simulink model "UticajSmetnji"  (R2014b)
settings: Solver=ode3  StartTime=0.0  StopTime=300  FixedStep=0.001  RelTol=1e-3
libraries: simulink x7
settings Model: Creator=Korisnik  LastModifiedBy=Korisnik

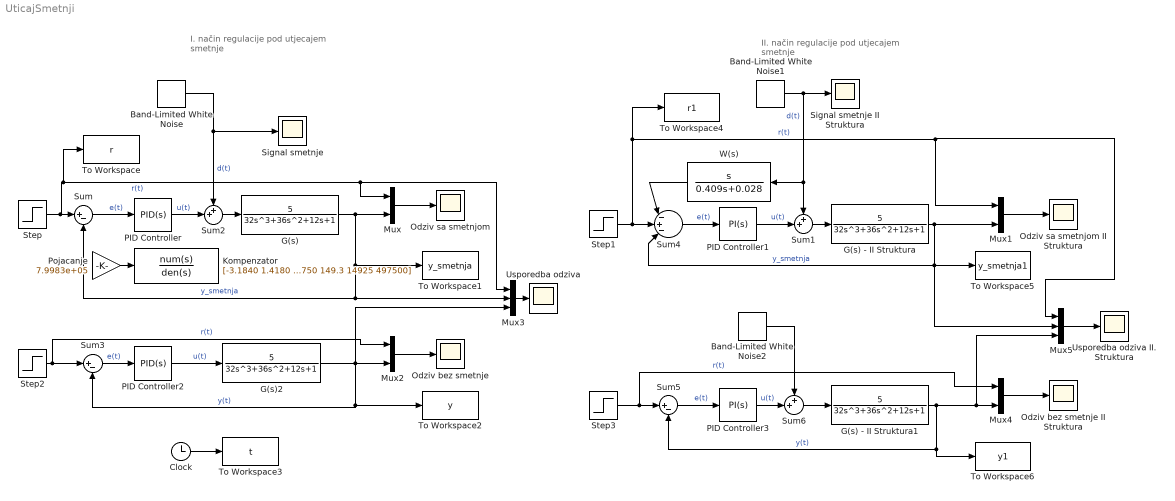
== system UticajSmetnji ==
  note: II. način regulacije pod utjecajem
      |                      smetnje
  note: I. način regulacije pod utjecajem
      |                     smetnje
  Band-Limited White Noise : simulink/Sources/Band-Limited White Noise  Cov=[0.001]  Ts=0.001  seed=[23341]
  Band-Limited White Noise1 : simulink/Sources/Band-Limited White Noise  Cov=[0.001]  Ts=0.001  seed=[23341]
  Band-Limited White Noise2 : simulink/Sources/Band-Limited White Noise  Cov=[0.001]  Ts=0.001  seed=[23341]
  Clock : Clock
  G(s) : TransferFcn  Numerator=[5]  Denominator=[32 36 12 1]
  G(s) - II Struktura : TransferFcn  Numerator=[5]  Denominator=[32 36 12 1]
  G(s) - II Struktura1 : TransferFcn  Numerator=[5]  Denominator=[32 36 12 1]
  G(s)2 : TransferFcn  Numerator=[5]  Denominator=[32 36 12 1]
  Kompenzator : TransferFcn  Numerator=[-3.1840 1.4180 1.0360 0.3980]  Denominator=[4.9750 149.3 14925 497500]
  Mux{,1..2,4} (4 alike) : Mux  Inputs=2
  Mux3 : Mux  Inputs=3
  Mux5 : Mux  Inputs=3
  Odziv bez smetnje : Scope
      settings: ShowLegends=on  SaveName=ScopeData2
  Odziv bez smetnje II Struktura : Scope
      settings: ShowLegends=on  SaveName=ScopeData6
  Odziv sa smetnjom : Scope
      settings: ShowLegends=on
  Odziv sa smetnjom II Struktura : Scope
      settings: ShowLegends=on
  PID Controller : simulink/Continuous/PID Controller  Controller=PID  TimeDomain=Continuous-time  SampleTime=-1  IntegratorMethod=Forward Euler  FilterMethod=Forward Euler  Form=Parallel  P=0.400421573227882  I=0.0460624565194868  D=0.464403326069187  N=2.07495559131807  InitialConditionSource=internal  InitialConditionForIntegrator=0  InitialConditionForFilter=0  ExternalReset=none  LimitOutput=off  UpperSaturationLimit=inf  LowerSaturationLimit=-inf  LinearizeAsGain=on  AntiWindupMode=none  Kb=1  TrackingMode=off  Kt=1  PParamMin=[]  PParamMax=[]  IParamMin=[]  IParamMax=[]  DParamMin=[]  DParamMax=[]  NParamMin=[]  NParamMax=[]  KbParamMin=[]  KbParamMax=[]  KtParamMin=[]  KtParamMax=[]  POutMin=[]  POutMax=[]  IOutMin=[]  IOutMax=[]  DOutMin=[]  DOutMax=[]  NOutMin=[]  NOutMax=[]  KbOutMin=[]  KbOutMax=[]  KtOutMin=[]  KtOutMax=[]  IntegratorOutMin=[]  IntegratorOutMax=[]  FilterOutMin=[]  FilterOutMax=[]  SumOutMin=[]  SumOutMax=[]  SumI1OutMin=[]  SumI1OutMax=[]  SumI2OutMin=[]  SumI2OutMax=[]  SumI3OutMin=[]  SumI3OutMax=[]  SumDOutMin=[]  SumDOutMax=[]  SaturationOutMin=[]  SaturationOutMax=[]  IntegratorContinuousStateAttributes=''  IntegratorStateMustResolveToSignalObject=off  IntegratorRTWStateStorageClass=Auto  FilterContinuousStateAttributes=''  FilterStateMustResolveToSignalObject=off  FilterRTWStateStorageClass=Auto  DifferentiatorICPrevScaledInput=0  DifferentiatorOutMin=[]  DifferentiatorOutMax=[]  UseFilter=on
  PID Controller1 : simulink/Continuous/PID Controller  Controller=PI  TimeDomain=Continuous-time  SampleTime=-1  IntegratorMethod=Forward Euler  FilterMethod=Forward Euler  Form=Parallel  P=0.409  I=0.028  D=0.464403326069187  N=2.07495559131807  InitialConditionSource=internal  InitialConditionForIntegrator=0  InitialConditionForFilter=0  ExternalReset=none  LimitOutput=off  UpperSaturationLimit=inf  LowerSaturationLimit=-inf  LinearizeAsGain=on  AntiWindupMode=none  Kb=1  TrackingMode=off  Kt=1  PParamMin=[]  PParamMax=[]  IParamMin=[]  IParamMax=[]  DParamMin=[]  DParamMax=[]  NParamMin=[]  NParamMax=[]  KbParamMin=[]  KbParamMax=[]  KtParamMin=[]  KtParamMax=[]  POutMin=[]  POutMax=[]  IOutMin=[]  IOutMax=[]  DOutMin=[]  DOutMax=[]  NOutMin=[]  NOutMax=[]  KbOutMin=[]  KbOutMax=[]  KtOutMin=[]  KtOutMax=[]  IntegratorOutMin=[]  IntegratorOutMax=[]  FilterOutMin=[]  FilterOutMax=[]  SumOutMin=[]  SumOutMax=[]  SumI1OutMin=[]  SumI1OutMax=[]  SumI2OutMin=[]  SumI2OutMax=[]  SumI3OutMin=[]  SumI3OutMax=[]  SumDOutMin=[]  SumDOutMax=[]  SaturationOutMin=[]  SaturationOutMax=[]  IntegratorContinuousStateAttributes=''  IntegratorStateMustResolveToSignalObject=off  IntegratorRTWStateStorageClass=Auto  FilterContinuousStateAttributes=''  FilterStateMustResolveToSignalObject=off  FilterRTWStateStorageClass=Auto  DifferentiatorICPrevScaledInput=0  DifferentiatorOutMin=[]  DifferentiatorOutMax=[]  UseFilter=on
  PID Controller2 : simulink/Continuous/PID Controller  Controller=PID  TimeDomain=Continuous-time  SampleTime=-1  IntegratorMethod=Forward Euler  FilterMethod=Forward Euler  Form=Parallel  P=0.400421573227882  I=0.0460624565194868  D=0.464403326069187  N=2.07495559131807  InitialConditionSource=internal  InitialConditionForIntegrator=0  InitialConditionForFilter=0  ExternalReset=none  LimitOutput=off  UpperSaturationLimit=inf  LowerSaturationLimit=-inf  LinearizeAsGain=on  AntiWindupMode=none  Kb=1  TrackingMode=off  Kt=1  PParamMin=[]  PParamMax=[]  IParamMin=[]  IParamMax=[]  DParamMin=[]  DParamMax=[]  NParamMin=[]  NParamMax=[]  KbParamMin=[]  KbParamMax=[]  KtParamMin=[]  KtParamMax=[]  POutMin=[]  POutMax=[]  IOutMin=[]  IOutMax=[]  DOutMin=[]  DOutMax=[]  NOutMin=[]  NOutMax=[]  KbOutMin=[]  KbOutMax=[]  KtOutMin=[]  KtOutMax=[]  IntegratorOutMin=[]  IntegratorOutMax=[]  FilterOutMin=[]  FilterOutMax=[]  SumOutMin=[]  SumOutMax=[]  SumI1OutMin=[]  SumI1OutMax=[]  SumI2OutMin=[]  SumI2OutMax=[]  SumI3OutMin=[]  SumI3OutMax=[]  SumDOutMin=[]  SumDOutMax=[]  SaturationOutMin=[]  SaturationOutMax=[]  IntegratorContinuousStateAttributes=''  IntegratorStateMustResolveToSignalObject=off  IntegratorRTWStateStorageClass=Auto  FilterContinuousStateAttributes=''  FilterStateMustResolveToSignalObject=off  FilterRTWStateStorageClass=Auto  DifferentiatorICPrevScaledInput=0  DifferentiatorOutMin=[]  DifferentiatorOutMax=[]  UseFilter=on
  PID Controller3 : simulink/Continuous/PID Controller  Controller=PI  TimeDomain=Continuous-time  SampleTime=-1  IntegratorMethod=Forward Euler  FilterMethod=Forward Euler  Form=Parallel  P=0.409  I=0.028  D=0.464403326069187  N=2.07495559131807  InitialConditionSource=internal  InitialConditionForIntegrator=0  InitialConditionForFilter=0  ExternalReset=none  LimitOutput=off  UpperSaturationLimit=inf  LowerSaturationLimit=-inf  LinearizeAsGain=on  AntiWindupMode=none  Kb=1  TrackingMode=off  Kt=1  PParamMin=[]  PParamMax=[]  IParamMin=[]  IParamMax=[]  DParamMin=[]  DParamMax=[]  NParamMin=[]  NParamMax=[]  KbParamMin=[]  KbParamMax=[]  KtParamMin=[]  KtParamMax=[]  POutMin=[]  POutMax=[]  IOutMin=[]  IOutMax=[]  DOutMin=[]  DOutMax=[]  NOutMin=[]  NOutMax=[]  KbOutMin=[]  KbOutMax=[]  KtOutMin=[]  KtOutMax=[]  IntegratorOutMin=[]  IntegratorOutMax=[]  FilterOutMin=[]  FilterOutMax=[]  SumOutMin=[]  SumOutMax=[]  SumI1OutMin=[]  SumI1OutMax=[]  SumI2OutMin=[]  SumI2OutMax=[]  SumI3OutMin=[]  SumI3OutMax=[]  SumDOutMin=[]  SumDOutMax=[]  SaturationOutMin=[]  SaturationOutMax=[]  IntegratorContinuousStateAttributes=''  IntegratorStateMustResolveToSignalObject=off  IntegratorRTWStateStorageClass=Auto  FilterContinuousStateAttributes=''  FilterStateMustResolveToSignalObject=off  FilterRTWStateStorageClass=Auto  DifferentiatorICPrevScaledInput=0  DifferentiatorOutMin=[]  DifferentiatorOutMax=[]  UseFilter=on
  Pojacanje : Gain  Gain=7.9983e+05
  Signal smetnje : Scope
      settings: ShowLegends=on  SaveName=ScopeData4
  Signal smetnje II Struktura : Scope
      settings: ShowLegends=on  SaveName=ScopeData5
  Step{,1..3} (4 alike) : Step  Time=0  SampleTime=0
  Sum : Sum  Inputs=|+-
  Sum1 : Sum  Inputs=++|
  Sum2 : Sum  Inputs=++|
  Sum3 : Sum  Inputs=|+-
  Sum4 : Sum  Inputs=|-+-|
  Sum5 : Sum  Inputs=|+-
  Sum6 : Sum  Inputs=++|
  To Workspace : ToWorkspace  VariableName=r  SampleTime=-1
  To Workspace1 : ToWorkspace  VariableName=y_smetnja  SampleTime=-1
  To Workspace2 : ToWorkspace  VariableName=y  SampleTime=-1
  To Workspace3 : ToWorkspace  VariableName=t  SampleTime=-1
  To Workspace4 : ToWorkspace  VariableName=r1  SampleTime=-1
  To Workspace5 : ToWorkspace  VariableName=y_smetnja1  SampleTime=-1
  To Workspace6 : ToWorkspace  VariableName=y1  SampleTime=-1
  Usporedba odziva : Scope
      settings: ShowLegends=on  SaveName=ScopeData3
  Usporedba odziva II. Struktura : Scope
      settings: ShowLegends=on  SaveName=ScopeData7
  W(s) : TransferFcn  Numerator=[1 0]  Denominator=[0.409 0.028]
  wires:
  Sum/1 -> PID Controller/1  "e(t)"
  Step/1 -> To Workspace/1, Mux3/1, Mux/1, Sum/1  "r(t)"
  G(s)/1 -> Sum/2, Mux3/2, To Workspace1/1, Mux/2  "y_smetnja"
  Mux/1 -> Odziv sa smetnjom/1
  Sum2/1 -> G(s)/1
  PID Controller/1 -> Sum2/2  "u(t)"
  Sum3/1 -> PID Controller2/1  "e(t)"
  Step2/1 -> Sum3/1, Mux2/1  "r(t)"
  G(s)2/1 -> Mux3/3, Sum3/2, To Workspace2/1, Mux2/2  "y(t)"
  Mux2/1 -> Odziv bez smetnje/1
  PID Controller2/1 -> G(s)2/1  "u(t)"
  Mux3/1 -> Usporedba odziva/1
  Clock/1 -> To Workspace3/1
  Band-Limited White Noise/1 -> Sum2/1, Signal smetnje/1  "d(t)"
  Pojacanje/1 -> Kompenzator/1
  Band-Limited White Noise1/1 -> W(s)/1, Sum1/1, Signal smetnje II Struktura/1  "d(t)"
  PID Controller1/1 -> Sum1/2  "u(t)"
  Sum1/1 -> G(s) - II Struktura/1
  Sum4/1 -> PID Controller1/1  "e(t)"
  G(s) - II Struktura/1 -> Mux5/2, Sum4/3, To Workspace5/1, Mux1/2  "y_smetnja"
  Mux1/1 -> Odziv sa smetnjom II Struktura/1
  Step1/1 -> Mux5/1, Mux1/1, To Workspace4/1, Sum4/2  "r(t)"
  W(s)/1 -> Sum4/1
  Step3/1 -> Mux4/1, Sum5/1  "r(t)"
  Sum5/1 -> PID Controller3/1  "e(t)"
  G(s) - II Struktura1/1 -> To Workspace6/1, Sum5/2, Mux5/3, Mux4/2  "y(t)"
  Mux4/1 -> Odziv bez smetnje II Struktura/1
  Mux5/1 -> Usporedba odziva II. Struktura/1
  Sum6/1 -> G(s) - II Struktura1/1
  PID Controller3/1 -> Sum6/2  "u(t)"
  Band-Limited White Noise2/1 -> Sum6/1
